simulink model "HW2SVPWM"  (R2024b)
settings: Solver=VariableStepAuto  StartTime=0.0  StopTime=1.0  MaxStep=10e-6  RelTol=1e-3
libraries: spsMeanLib x7, spsMosfetLib x6, simulink x3, spsTHDLib x2, spsCurrentMeasurementLib x1, spsDCVoltageSourceLib x1, spsGroundLib x1, spsTriangleGeneratorLib x1, spsThreePhaseSeriesRLCBranchLib x1, spsThreePhaseVIMeasurementLib x1, spsVoltageMeasurementLib x1, sps_lib x1
settings Model: Creator=joekr  LastModifiedBy=joekr

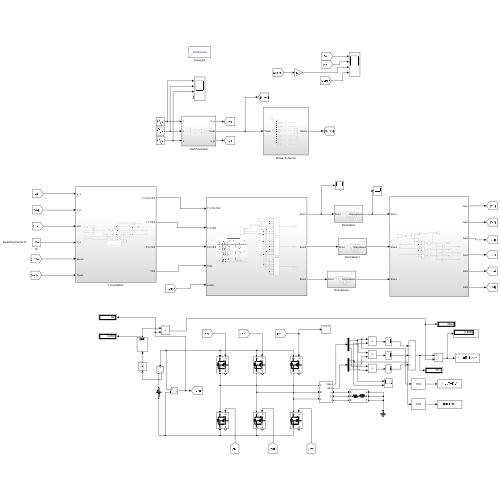
[thumbnail: Simulink's stored preview of the top-level diagram]
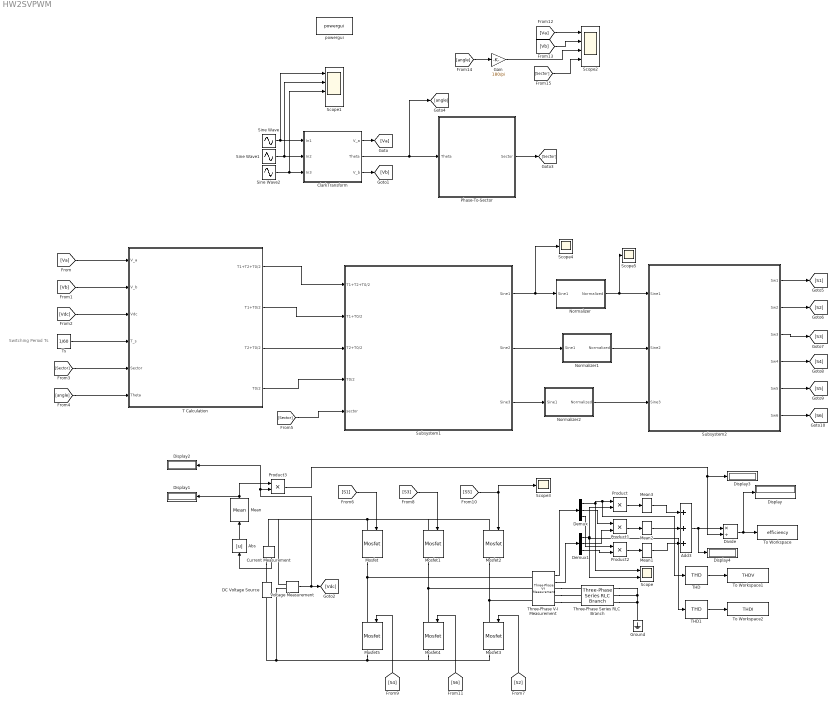
== system HW2SVPWM ==
  note: Switching Period Ts
  Abs : Abs  SaturateOnIntegerOverflow=off
  Add3 : Sum  Inputs=+++
  ClarkTransform : Subsystem
  Current Measurement : spsCurrentMeasurementLib/Current Measurement  PhasorSimulation=off  OutputType=Complex  PSBequivalent=0
  DC Voltage Source : spsDCVoltageSourceLib/DC Voltage Source  Amplitude=400  Measurements=None
  Demux : Demux  Outputs=3
  Demux1 : Demux  Outputs=3
  Display{,1..4} (5 alike) : Display
  Divide : Product  Inputs=*/
  Gain : Gain  Gain=180/pi
  Ground : spsGroundLib/Ground  LConnTagsString=a
  Mean{,1..3} (4 alike) : spsMeanLib/Mean  Freq=60  Vinit=0  Ts=0
  Mosfet{,1..5} (6 alike) : spsMosfetLib/Mosfet  Ron=0.1  Lon=0  Rd=0.01  Vfd=0  IC=0  Rs=1e5  Cs=inf  Measurements=on
  Normalizer : Subsystem
  Normalizer1 : Subsystem
  Normalizer2 : Subsystem
  Phase-To-Sector : Subsystem
  Product{,1..3} (4 alike) : Product
  Scope : Scope  NumInputPorts=2
  Scope1 : Scope  NumInputPorts=4
  Scope2 : Scope  NumInputPorts=4
  Scope3 : Scope
  Scope4 : Scope
  Scope5 : Scope
  Sine Wave : Sin  Frequency=120*pi  SampleTime=0
  Sine Wave1 : Sin  Frequency=120*pi  Phase=2*pi/3  SampleTime=0
  Sine Wave2 : Sin  Frequency=120*pi  Phase=4*pi/3  SampleTime=0
  Subsystem1 : Subsystem
  Subsystem2 : Subsystem
  T Calculation : Subsystem
  THD : spsTHDLib/THD  Freq=60  Ts=0
  THD1 : spsTHDLib/THD  Freq=60  Ts=0
  Three-Phase Series RLC Branch : spsThreePhaseSeriesRLCBranchLib/Three-Phase Series RLC Branch  LConnTagsString=A|B|C  RConnTagsString=A|B|C  BranchType=RL  Resistance=100  Inductance=0.1  Capacitance=1e-6  Measurements=None
  Three-Phase V-I Measurement : spsThreePhaseVIMeasurementLib/Three-Phase V-I Measurement  VoltageMeasurement=phase-to-ground  SetLabelV=off  LabelV=Vabc  Vpu=off  VpuLL=off  CurrentMeasurement=yes  SetLabelI=off  LabelI=Iabc  Ipu=off  Pbase=100e6  Vbase=500e3  OutputType=Complex  PhasorSimulation=off  PSBequivalent=0
  To Workspace : ToWorkspace  VariableName=efficiency  SaveFormat=Structure With Time  SampleTime=-1
  To Workspace1 : ToWorkspace  VariableName=THDV  SaveFormat=Structure With Time  SampleTime=-1
  To Workspace2 : ToWorkspace  VariableName=THDI  SaveFormat=Structure With Time  SampleTime=-1
  Ts : Constant  Value=1/60
  Voltage Measurement : spsVoltageMeasurementLib/Voltage Measurement  PhasorSimulation=off  OutputType=Complex  PSBequivalent=0
  powergui : sps_lib/powergui  Priority=1  SimulationMode=Continuous  SampleTime=50e-6  frequency=60  Iterations=50  frequencyindice=0  Pbase=100e6  ErrMax=1e-4  UnitsV=kV  UnitsW=MW  buscounter=0  FunctionMessages=off  echomessages=off  EnableUseOfTLC=off  CurrentSourceSwitches=off  DisableSnubberDevices=off  DisableRonSwitches=off  DisableVfSwitches=off  DisplayEquations=off  AutomaticDiscreteSolvers=off  SolverType=Tustin/Backward Euler (TBE)  Interpol=off  ExternalGateDelay=off  methode=off  Ts=100  x0status=blocks  SPID=on  SwTol=0  HookPort=off  NonlinearTolerance=1e-4  nMaxIteration=100  ContinueOnMaxIteration=off  RestoreLinks=warning  ResistiveCurrentMeasurement=off  Frange=[0:2:500]  Ylog=off  Xlog=on  ShowGrid=off  save=off  variable=ZData  structure=0  ZoomFFT=off  StartTime=0.0  cycles=1  DisplayStyle=1  fundamental=60  FreqAxis=off  MaxFrequency=1000  frequencyindicesteady=1  RmsSteady=1  display=off
  wires:
  Sine Wave/1 -> Scope1/1, ClarkTransform/1(In1)
  Sine Wave1/1 -> Scope1/2, ClarkTransform/2(In2)
  Sine Wave2/1 -> Scope1/3, ClarkTransform/3(In3)
  ClarkTransform/2(Theta) -> [angle], Phase-To-Sector/1(Theta)
  ClarkTransform/1(V_a) -> [Va]
  ClarkTransform/3(V_b) -> [Vb]
  Voltage Measurement/1 -> Display2/1, Product3/2, [Vdc]
  Phase-To-Sector/1(Sector) -> [Sector]
  [Va] -> T Calculation/1(V_a)
  [Vb] -> T Calculation/2(V_b)
  [Vdc] -> T Calculation/3(Vdc)
  Ts/1 -> T Calculation/4(T_s)
  [Sector] -> T Calculation/5(Sector)
  [angle] -> T Calculation/6(Theta)
  T Calculation/1(T1+T2+T0/2) -> Subsystem1/1(T1+T2+T0/2)
  T Calculation/2(T1+T0/2) -> Subsystem1/2(T1+T0/2)
  T Calculation/4(T0/2) -> Subsystem1/4(T0/2)
  T Calculation/3(T2+T0/2) -> Subsystem1/3(T2+T0/2)
  [Sector] -> Subsystem1/5(sector)
  Subsystem2/1(Sw1) -> [S1]
  Subsystem2/2(Sw2) -> [S2]
  Subsystem2/3(Sw3) -> [S3]
  Subsystem2/4(Sw4) -> [S4]
  Subsystem2/5(Sw5) -> [S5]
  Subsystem2/6(Sw6) -> [S6]
  [S1] -> Mosfet/1
  [S2] -> Mosfet3/1
  [S3] -> Mosfet1/1
  [S4] -> Mosfet5/1
  [S5] -> Mosfet2/1, Scope3/1
  [S6] -> Mosfet4/1
  Three-Phase V-I Measurement/1 -> Demux/1
  Three-Phase V-I Measurement/2 -> Demux1/1
  [Va] -> Scope2/1
  [Vb] -> Scope2/2
  [Sector] -> Scope2/4
  [angle] -> Gain/1
  Gain/1 -> Scope2/3
  Subsystem1/1(Sine1) -> Scope4/1, Normalizer/1(Sine1)
  Normalizer/1(Normalized) -> Scope5/1, Subsystem2/1(Sine1)
  Normalizer1/1(Normalized) -> Subsystem2/2(Sine2)
  Normalizer2/1(Normalized) -> Subsystem2/3(Sine3)
  Demux/1 -> Scope/1, THD/1, Product/1
  Demux/2 -> Product1/1
  Demux1/1 -> Scope/2, THD1/1, Product/2
  Demux/3 -> Product2/1
  Demux1/2 -> Product1/2
  Demux1/3 -> Product2/2
  Product2/1 -> Mean1/1
  Product1/1 -> Mean2/1
  Product/1 -> Mean3/1
  Mean2/1 -> Add3/2
  Mean3/1 -> Add3/1
  Mean1/1 -> Add3/3
  Add3/1 -> Display4/1, Divide/1
  Abs/1 -> Mean/1
  Current Measurement/1 -> Abs/1
  Mean/1 -> Product3/1, Display1/1
  Product3/1 -> Display3/1, Divide/2
  Divide/1 -> Display/1, To Workspace/1
  THD1/1 -> To Workspace2/1
  THD/1 -> To Workspace1/1
  Subsystem1/2(Sine2) -> Normalizer1/1(Sine1)
  Subsystem1/3(Sine3) -> Normalizer2/1(Sine1)
  connections:
  Mosfet/RConn1 -- Three-Phase V-I Measurement/LConn1 -- Mosfet5/LConn1
  Mosfet1/RConn1 -- Three-Phase V-I Measurement/LConn2 -- Mosfet4/LConn1
  Mosfet2/RConn1 -- Three-Phase V-I Measurement/LConn3 -- Mosfet3/LConn1
  Three-Phase V-I Measurement/RConn1 -- Three-Phase Series RLC Branch/LConn1
  Three-Phase V-I Measurement/RConn2 -- Three-Phase Series RLC Branch/LConn2
  Three-Phase V-I Measurement/RConn3 -- Three-Phase Series RLC Branch/LConn3
  Mosfet/LConn1 -- Current Measurement/LConn1 -- Voltage Measurement/LConn1 -- Mosfet2/LConn1 -- Mosfet1/LConn1
  Mosfet5/RConn1 -- Mosfet3/RConn1 -- Mosfet4/RConn1 -- Voltage Measurement/LConn2 -- DC Voltage Source/LConn1
  Three-Phase Series RLC Branch/RConn1 -- Three-Phase Series RLC Branch/RConn3 -- Ground/LConn1 -- Three-Phase Series RLC Branch/RConn2
  Current Measurement/RConn1 -- DC Voltage Source/RConn1

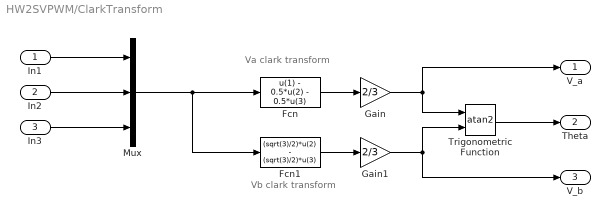
== system HW2SVPWM/ClarkTransform ==
  note: Vb clark transform
  note: Va clark transform
  In1 : Inport
  In2 : Inport  Port=2
  In3 : Inport  Port=3
  Fcn : Fcn  Expr=u(1) - 0.5*u(2) - 0.5*u(3)
  Fcn1 : Fcn  Expr=(sqrt(3)/2)*u(2) - (sqrt(3)/2)*u(3)
  Gain : Gain  Gain=2/3
  Gain1 : Gain  Gain=2/3
  Mux : Mux  Inputs=3
  Trigonometric Function : Trigonometry  Operator=atan2
  V_a : Outport
  Theta : Outport  Port=2
  V_b : Outport  Port=3
  wires:
  Trigonometric Function/1 -> Theta/1
  Gain/1 -> Trigonometric Function/1, V_a/1
  Gain1/1 -> Trigonometric Function/2, V_b/1
  Mux/1 -> Fcn1/1, Fcn/1
  Fcn/1 -> Gain/1
  In2/1 -> Mux/2
  Fcn1/1 -> Gain1/1
  In3/1 -> Mux/3
  In1/1 -> Mux/1

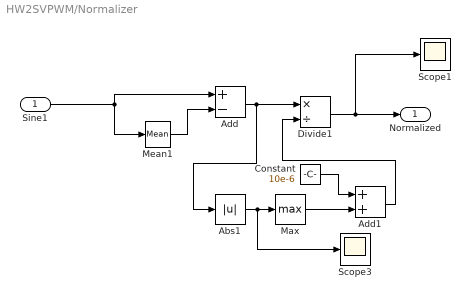
== system HW2SVPWM/Normalizer ==
  Sine1 : Inport
  Abs1 : Abs  SaturateOnIntegerOverflow=off
  Add : Sum  Inputs=+-
  Add1 : Sum
  Constant : Constant  Value=10e-6
  Divide1 : Product  Inputs=*/
  Max : MinMax  Function=max
  Mean1 : spsMeanLib/Mean  Freq=60  Vinit=0  Ts=0
  Scope1 : Scope
  Scope3 : Scope
  Normalized : Outport
  wires:
  Sine1/1 -> Add/1, Mean1/1
  Mean1/1 -> Add/2
  Divide1/1 -> Scope1/1, Normalized/1
  Add/1 -> Abs1/1, Divide1/1
  Abs1/1 -> Scope3/1, Max/1
  Max/1 -> Add1/2
  Add1/1 -> Divide1/2
  Constant/1 -> Add1/1

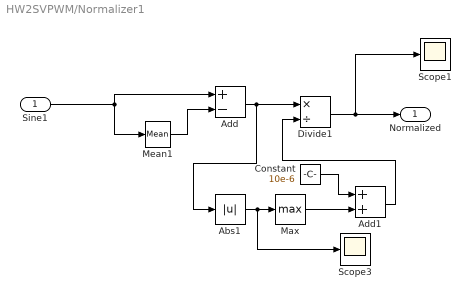
== system HW2SVPWM/Normalizer1 ==
  Sine1 : Inport
  Abs1 : Abs  SaturateOnIntegerOverflow=off
  Add : Sum  Inputs=+-
  Add1 : Sum
  Constant : Constant  Value=10e-6
  Divide1 : Product  Inputs=*/
  Max : MinMax  Function=max
  Mean1 : spsMeanLib/Mean  Freq=60  Vinit=0  Ts=0
  Scope1 : Scope
  Scope3 : Scope
  Normalized : Outport
  wires:
  Sine1/1 -> Add/1, Mean1/1
  Mean1/1 -> Add/2
  Divide1/1 -> Scope1/1, Normalized/1
  Add/1 -> Abs1/1, Divide1/1
  Abs1/1 -> Scope3/1, Max/1
  Max/1 -> Add1/2
  Add1/1 -> Divide1/2
  Constant/1 -> Add1/1

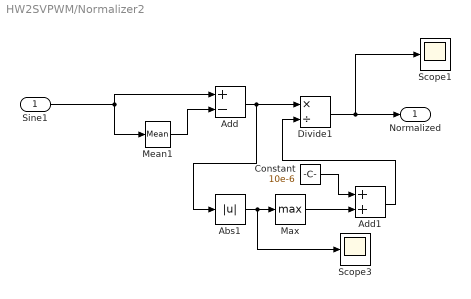
== system HW2SVPWM/Normalizer2 ==
  Sine1 : Inport
  Abs1 : Abs  SaturateOnIntegerOverflow=off
  Add : Sum  Inputs=+-
  Add1 : Sum
  Constant : Constant  Value=10e-6
  Divide1 : Product  Inputs=*/
  Max : MinMax  Function=max
  Mean1 : spsMeanLib/Mean  Freq=60  Vinit=0  Ts=0
  Scope1 : Scope
  Scope3 : Scope
  Normalized : Outport
  wires:
  Sine1/1 -> Add/1, Mean1/1
  Mean1/1 -> Add/2
  Divide1/1 -> Scope1/1, Normalized/1
  Add/1 -> Abs1/1, Divide1/1
  Abs1/1 -> Scope3/1, Max/1
  Max/1 -> Add1/2
  Add1/1 -> Divide1/2
  Constant/1 -> Add1/1

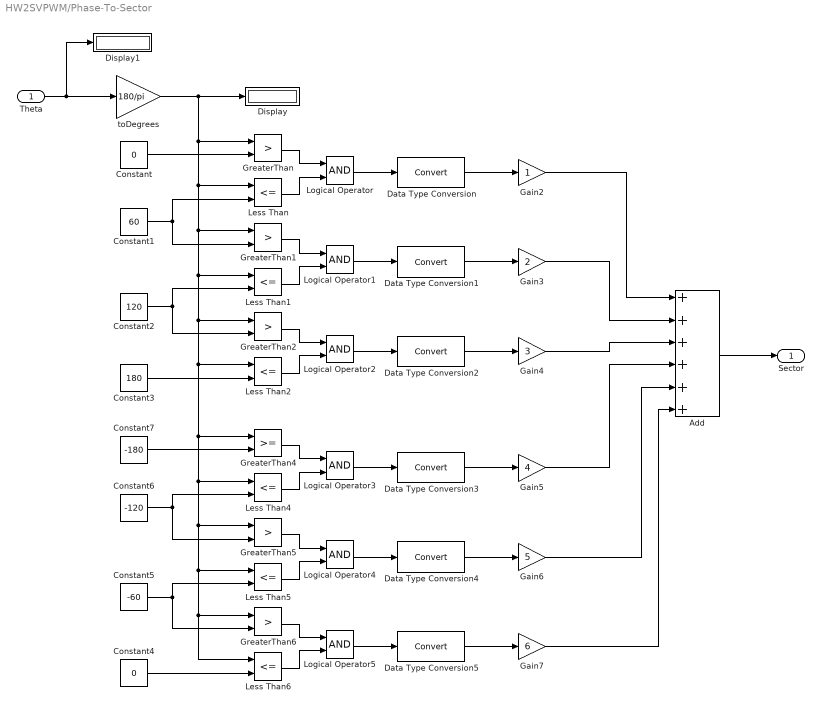
== system HW2SVPWM/Phase-To-Sector ==
  Theta : Inport
  Add : Sum  Inputs=++++++
  Constant : Constant  Value=0
  Constant1 : Constant  Value=60
  Constant2 : Constant  Value=120
  Constant3 : Constant  Value=180
  Constant4 : Constant  Value=0
  Constant5 : Constant  Value=-60
  Constant6 : Constant  Value=-120
  Constant7 : Constant  Value=-180
  Data Type Conversion{,1..5} (6 alike) : DataTypeConversion  SaturateOnIntegerOverflow=off  RndMeth=Floor
  Display : Display
  Display1 : Display
  Gain2 : Gain
  Gain3 : Gain  Gain=2
  Gain4 : Gain  Gain=3
  Gain5 : Gain  Gain=4
  Gain6 : Gain  Gain=5
  Gain7 : Gain  Gain=6
  GreaterThan{,1..2,5..6} (5 alike) : RelationalOperator  Operator=>  OutDataTypeStr=boolean  RndMeth=Simplest  InputSameDT=off
  GreaterThan4 : RelationalOperator  OutDataTypeStr=boolean  RndMeth=Simplest  InputSameDT=off
  Less Than{,1..2,4..6} (6 alike) : RelationalOperator  Operator=<=  OutDataTypeStr=boolean  RndMeth=Simplest  InputSameDT=off
  Logical Operator{,1..5} (6 alike) : Logic  AllPortsSameDT=off  OutDataTypeStr=boolean
  toDegrees : Gain  Gain=180/pi
  Sector : Outport
  wires:
  Constant6/1 -> Less Than4/2, GreaterThan5/2
  GreaterThan4/1 -> Logical Operator3/1
  Gain5/1 -> Add/4
  Logical Operator3/1 -> Data Type Conversion3/1
  toDegrees/1 -> Display/1, Less Than6/1, GreaterThan6/1, Less Than5/1, GreaterThan5/1, Less Than4/1, GreaterThan4/1, Less Than2/1, GreaterThan2/1, Less Than1/1, GreaterThan1/1, Less Than/1, GreaterThan/1
  Gain7/1 -> Add/6
  Constant1/1 -> Less Than/2, GreaterThan1/2
  Gain2/1 -> Add/1
  Less Than6/1 -> Logical Operator5/2
  Logical Operator4/1 -> Data Type Conversion4/1
  Constant4/1 -> Less Than6/2
  Logical Operator5/1 -> Data Type Conversion5/1
  GreaterThan6/1 -> Logical Operator5/1
  Less Than5/1 -> Logical Operator4/2
  Less Than4/1 -> Logical Operator3/2
  GreaterThan5/1 -> Logical Operator4/1
  Less Than1/1 -> Logical Operator1/2
  Constant3/1 -> Less Than2/2
  Logical Operator/1 -> Data Type Conversion/1
  Logical Operator2/1 -> Data Type Conversion2/1
  GreaterThan2/1 -> Logical Operator2/1
  Less Than2/1 -> Logical Operator2/2
  Data Type Conversion3/1 -> Gain5/1
  Constant2/1 -> GreaterThan2/2, Less Than1/2
  Theta/1 -> Display1/1, toDegrees/1
  Data Type Conversion1/1 -> Gain3/1
  GreaterThan1/1 -> Logical Operator1/1
  Gain6/1 -> Add/5
  Logical Operator1/1 -> Data Type Conversion1/1
  GreaterThan/1 -> Logical Operator/1
  Data Type Conversion5/1 -> Gain7/1
  Gain3/1 -> Add/2
  Add/1 -> Sector/1
  Constant/1 -> GreaterThan/2
  Constant5/1 -> Less Than5/2, GreaterThan6/2
  Constant7/1 -> GreaterThan4/2
  Less Than/1 -> Logical Operator/2
  Data Type Conversion4/1 -> Gain6/1
  Gain4/1 -> Add/3
  Data Type Conversion/1 -> Gain2/1
  Data Type Conversion2/1 -> Gain4/1

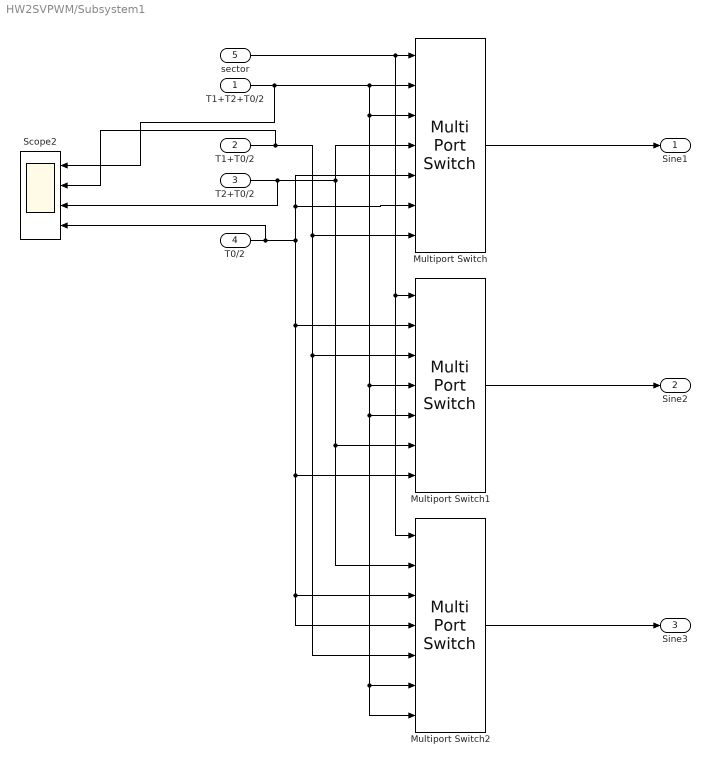
== system HW2SVPWM/Subsystem1 ==
  T1+T2+T0/2 : Inport
  T1+T0/2 : Inport  Port=2
  T2+T0/2 : Inport  Port=3
  T0/2 : Inport  Port=4
  sector : Inport  Port=5
  Multiport Switch : MultiPortSwitch  Inputs=6  SaturateOnIntegerOverflow=off  InputSameDT=off
  Multiport Switch1 : MultiPortSwitch  Inputs=6  SaturateOnIntegerOverflow=off  InputSameDT=off
  Multiport Switch2 : MultiPortSwitch  Inputs=6  SaturateOnIntegerOverflow=off  InputSameDT=off
  Scope2 : Scope  NumInputPorts=4
  Sine1 : Outport
  Sine2 : Outport  Port=2
  Sine3 : Outport  Port=3
  wires:
  T1+T2+T0/2/1 -> Scope2/1, Multiport Switch2/7, Multiport Switch2/6, Multiport Switch1/5, Multiport Switch1/4, Multiport Switch/3, Multiport Switch/2
  T1+T0/2/1 -> Scope2/2, Multiport Switch2/5, Multiport Switch1/3, Multiport Switch/7
  Multiport Switch2/1 -> Sine3/1
  sector/1 -> Multiport Switch2/1, Multiport Switch1/1, Multiport Switch/1
  T0/2/1 -> Scope2/4, Multiport Switch2/3, Multiport Switch2/4, Multiport Switch1/7, Multiport Switch1/2, Multiport Switch/6, Multiport Switch/5
  Multiport Switch/1 -> Sine1/1
  T2+T0/2/1 -> Scope2/3, Multiport Switch2/2, Multiport Switch1/6, Multiport Switch/4
  Multiport Switch1/1 -> Sine2/1

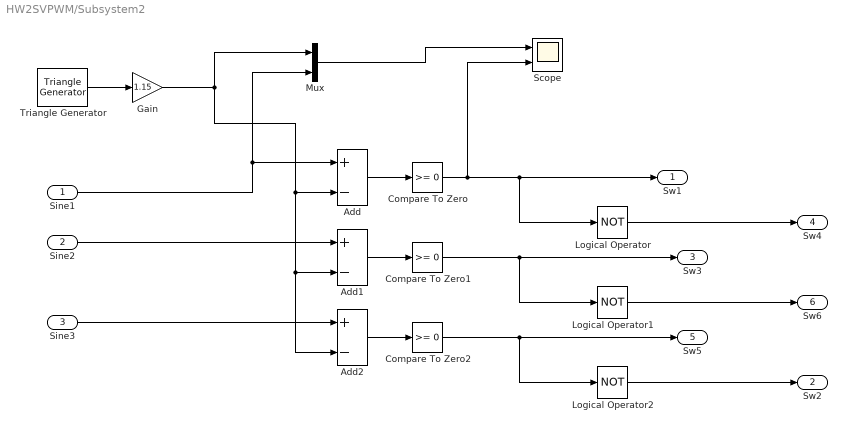
== system HW2SVPWM/Subsystem2 ==
  Sine1 : Inport
  Sine2 : Inport  Port=2
  Sine3 : Inport  Port=3
  Add : Sum  Inputs=+-
  Add1 : Sum  Inputs=+-
  Add2 : Sum  Inputs=+-
  Compare To Zero : simulink/Logic and Bit Operations/Compare To Zero  relop=>=  OutDataTypeStr=boolean
  Compare To Zero1 : simulink/Logic and Bit Operations/Compare To Zero  relop=>=  OutDataTypeStr=boolean
  Compare To Zero2 : simulink/Logic and Bit Operations/Compare To Zero  relop=>=  OutDataTypeStr=boolean
  Gain : Gain  Gain=1.15
  Logical Operator : Logic  Operator=NOT  AllPortsSameDT=off  OutDataTypeStr=boolean
  Logical Operator1 : Logic  Operator=NOT  AllPortsSameDT=off  OutDataTypeStr=boolean
  Logical Operator2 : Logic  Operator=NOT  AllPortsSameDT=off  OutDataTypeStr=boolean
  Mux : Mux  Inputs=2
  Scope : Scope  NumInputPorts=2
  Triangle Generator : spsTriangleGeneratorLib/Triangle Generator  Freq=600  Phase=0  Ts=0
  Sw1 : Outport
  Sw2 : Outport  Port=2
  Sw3 : Outport  Port=3
  Sw4 : Outport  Port=4
  Sw5 : Outport  Port=5
  Sw6 : Outport  Port=6
  wires:
  Logical Operator1/1 -> Sw6/1
  Compare To Zero2/1 -> Sw5/1, Logical Operator2/1
  Add/1 -> Compare To Zero/1
  Logical Operator/1 -> Sw4/1
  Sine1/1 -> Add/1, Mux/2
  Triangle Generator/1 -> Gain/1
  Logical Operator2/1 -> Sw2/1
  Compare To Zero1/1 -> Sw3/1, Logical Operator1/1
  Compare To Zero/1 -> Scope/2, Sw1/1, Logical Operator/1
  Add1/1 -> Compare To Zero1/1
  Add2/1 -> Compare To Zero2/1
  Mux/1 -> Scope/1
  Gain/1 -> Add2/2, Add1/2, Add/2, Mux/1
  Sine2/1 -> Add1/1
  Sine3/1 -> Add2/1

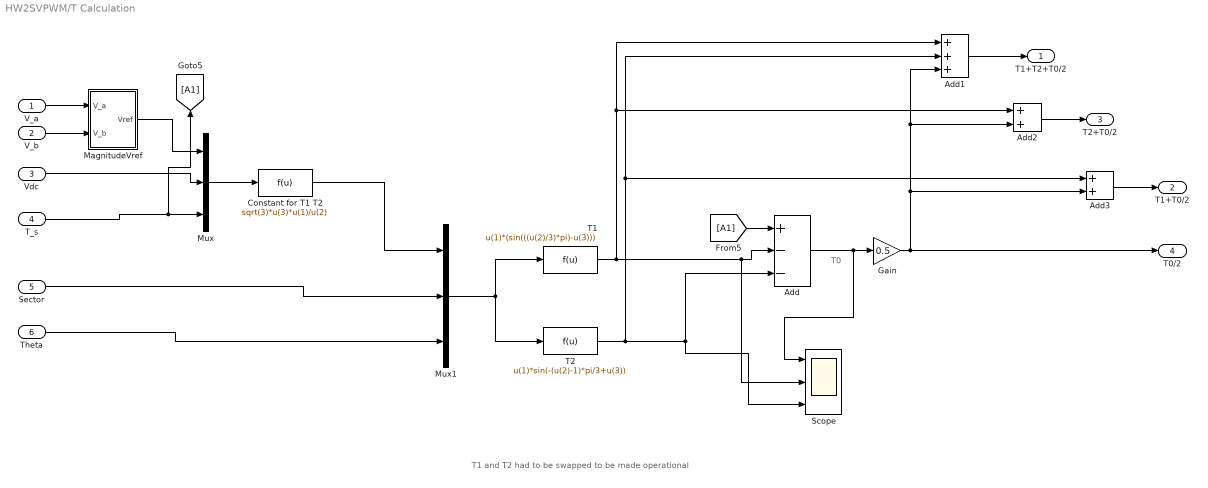
== system HW2SVPWM/T Calculation ==
  note: T1 and T2 had to be swapped to be made operational
  note: T0
  V_a : Inport
  V_b : Inport  Port=2
  Vdc : Inport  Port=3
  T_s : Inport  Port=4
  Sector : Inport  Port=5
  Theta : Inport  Port=6
  Add : Sum  Inputs=+--
  Add1 : Sum  Inputs=+++
  Add2 : Sum
  Add3 : Sum
  Constant for T1 T2 : Fcn  Expr=sqrt(3)*u(3)*u(1)/u(2)
  Gain : Gain  Gain=0.5
  MagnitudeVref : Subsystem
  Mux : Mux  Inputs=3
  Mux1 : Mux  Inputs=3
  Scope : Scope  NumInputPorts=3
  T1 : Fcn  Expr=u(1)*(sin(((u(2)/3)*pi)-u(3)))
  T2 : Fcn  Expr=u(1)*sin(-(u(2)-1)*pi/3+u(3))
  T1+T2+T0/2 : Outport
  T1+T0/2 : Outport  Port=2
  T2+T0/2 : Outport  Port=3
  T0/2 : Outport  Port=4
  wires:
  Vdc/1 -> Mux/2
  Mux/1 -> Constant for T1 T2/1
  T1/1 -> Add2/1, Add1/1, Scope/2, Add/2
  [A1] -> Add/1
  Sector/1 -> Mux1/2
  V_a/1 -> MagnitudeVref/1(V_a)
  T_s/1 -> [A1], Mux/3
  Mux1/1 -> T2/1, T1/1
  V_b/1 -> MagnitudeVref/2(V_b)
  T2/1 -> Add3/1, Add1/2, Scope/3, Add/3
  MagnitudeVref/1(Vref) -> Mux/1
  Theta/1 -> Mux1/3
  Gain/1 -> T0/2/1, Add3/2, Add2/2, Add1/3
  Constant for T1 T2/1 -> Mux1/1
  Add/1 -> Scope/1, Gain/1
  Add1/1 -> T1+T2+T0/2/1
  Add2/1 -> T2+T0/2/1
  Add3/1 -> T1+T0/2/1

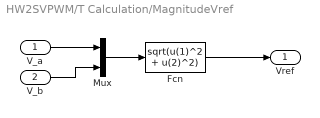
== system HW2SVPWM/T Calculation/MagnitudeVref ==
  V_a : Inport
  V_b : Inport  Port=2
  Fcn : Fcn  Expr=sqrt(u(1)^2 + u(2)^2)
  Mux : Mux  Inputs=2
  Vref : Outport
  wires:
  Mux/1 -> Fcn/1
  V_a/1 -> Mux/1
  V_b/1 -> Mux/2
  Fcn/1 -> Vref/1
